simulink model "TestSineSetPoint"  (R2016b)
settings: Solver=FixedStepAuto  StartTime=0.0  StopTime=inf  FixedStep=0.002  RelTol=1e-3
settings Model: Creator=march  LastModifiedBy=march

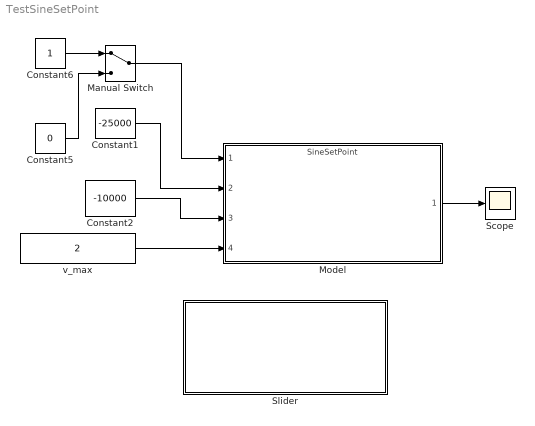
== system TestSineSetPoint ==
  Constant1 : Constant  Value=-25000
  Constant2 : Constant  Value=-10000
  Constant5 : Constant  Value=0
  Constant6 : Constant
  Manual Switch : ManualSwitch
  Model : ModelReference  ModelNameDialog=SineSetPoint  SimulationMode=Normal  ModelReferenceVersion=1.24
  Scope : Scope
  Slider : Subsystem  DialogController=hmiCreateDDGDialog  IsWebBlock=on  mask(MWDashboardBlock){webBlockId=86a9a32f-bde2-45b6-9ae7-0381a700462c, webBlockType=slider, ShowInLibBrowser=on, ShowInitialText=on, HMISrcModelName=TestSineSetPoint}
      mask prompts: webBlockId "WebBlock Id"; webBlockType "WebBlock Type"; HMISrcModelName "Source Model"
      mask help: SimulinkHMI:dialogs:SliderDialogDesc
      mask Help: helpview([docroot '/mapfiles/simulink.map'], 'hmi_slider')
      mask Display:
      | if strcmp(get_param(bdroot(gcb),'BlockDiagramType'), 'library')
      |     image([(matlabroot) '/toolbox/simulink/hmi/icons/Slider.png']);
      | end
  v_max : Constant  Value=2
  wires:
  Model/1 -> Scope/1
  Manual Switch/1 -> Model/1
  Constant1/1 -> Model/2
  Constant2/1 -> Model/3
  v_max/1 -> Model/4
  Constant5/1 -> Manual Switch/2
  Constant6/1 -> Manual Switch/1

== system TestSineSetPoint/Slider ==
